simulink model "CRTsfun"  (Simulink 8.0)
settings: Solver=ode45  StartTime=0.0  StopTime=10.0  RelTol=1e-3
undefined symbols (not defined in the file or in its folder): vicrt_initcallback, vicrt_initmexcallback, vicrt_inputfile, vicrt_simulationmanager
(part 1 of 3)
settings Model: Creator=battags  LastModifiedBy=battags

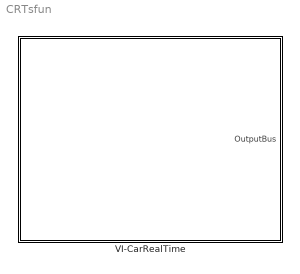
== system CRTsfun ==
  VI-CarRealTime : Subsystem  InitFcn=vicrt_simulationmanager(0);
      mask help: Full VI-CarRealTime mex integrated with IO Bus
      settings: CopyFcn=set_param(gcb, 'LinkStatus', 'none');  ModelCloseFcn=vicrt_simulationmanager(2);  OpenFcn=vicrt_simulationmanager(1);
      mask Display: image(imread('vehicle.jpg'));color('red');port_label('output',1,'OutputBus');

== system CRTsfun/VI-CarRealTime ==
  Input_Bus : Subsystem  LoadFcn=vicrt_initcallback(gcb);
      settings: CopyFcn=vicrt_initcallback(gcb);
  Output_Bus : Subsystem  Description=Outputs
      settings: CopyFcn=%set_param(gcb, 'LinkStatus', 'none')
  vicrt_mex Standard : Subsystem  mask{vicrt_inputfile=vicrt_inputfile, vicrt_outprefix='', intStep=0.001, AniFlag=off, inpPortDim=225, outPortDim=1100}
      mask prompts: vicrt_inputfile "VI-CarRealtime input file"; vicrt_outprefix "VI-CarRealTime output prefix"; intStep "Integration step"; AniFlag "live animation"; inpPortDim "input port dimension"; outPortDim "output port dimension"
      mask init:
      | custDriv=[1,1,1];
      settings: CopyFcn=set_param(gcb, 'LinkStatus', 'none')
  OutputBus : Outport
  wires:
  Output_Bus/1(OutputBus) -> OutputBus/1
  Input_Bus/1(vicrt input) -> vicrt_mex Standard/1(In1)
  vicrt_mex Standard/1(Out1) -> Output_Bus/1(Outputs)

== system CRTsfun/VI-CarRealTime/Input_Bus ==
  Bus2Map : Subsystem
  Inputs : Subsystem
  Standard_Input_Bus : Constant
  VicrtBusAssignment : BusAssignment  AssignedSignals=Standard_Input_Bus
  vicrt input : Outport
  wires:
  Standard_Input_Bus/1 -> VicrtBusAssignment/2
  Inputs/1(Inputs) -> VicrtBusAssignment/1  "Inputs"
  VicrtBusAssignment/1 -> Bus2Map/1(Bus In)
  Bus2Map/1(Map Out) -> vicrt input/1

== system CRTsfun/VI-CarRealTime/Output_Bus ==
  Outputs : Inport
  IOmap2bus : Subsystem
  VicrtBusSelector : BusSelector  InitFcn=warning('off','Simulink:blocks:BusSelectorDuplicateLeafSignalInMuxedOutput');  StartFcn=warning('on','Simulink:blocks:BusSelectorDuplicateLeafSignalInMuxedOutput');  OutputSignals=aero_forces  OutputAsBus=on
  adapter : Subsystem
  OutputBus : Outport
  wires:
  adapter/1(outputBus) -> OutputBus/1
  VicrtBusSelector/1 -> adapter/1(inputBus)
  Outputs/1 -> IOmap2bus/1(In)
  IOmap2bus/1(Out) -> VicrtBusSelector/1

== system CRTsfun/VI-CarRealTime/vicrt_mex Standard ==
  In1 : Inport
  vicrt_mex : S-Function  InitFcn=vicrt_initmexcallback(gcb);  FunctionName=vicrt_mex  Parameters=vicrt_inputfile,vicrt_outprefix,AniFlag,intStep,inpPortDim,outPortDim  EnableBusSupport=off
  Out1 : Outport
  wires:
  In1/1 -> vicrt_mex/1
  vicrt_mex/1 -> Out1/1

== system CRTsfun/VI-CarRealTime/Input_Bus/Bus2Map ==
  Bus In : Inport
  Bus Selector : BusSelector  OutputSignals=Driver_Demands.str_swa,Driver_Demands.throttle,Driver_Demands.gear,Driver_Demands.clutch,Driver_Demands.brake,Driver_Demands.rack_displacement,Brake_System_General.brk_mast_cyl_pres,Brake_System_General.brk_bias_front,Driver_Demands.user_maneuver_ID,Friction.tire_mu.L1,Friction.tire_mu.L2,Friction.tire_mu.R1,Friction.tire_mu.R2,Subsystem_Activation.Internal_Brake_System_Activity.L1,Brake_System.brk_mmag_sign.L1,Brake_System.brk_mmag_unsign.L1,Brake_System.brk_pres.L1,Brake_System.brk_pres_gain.L1,Brake_System.brk_mu.L1,Subsystem_Activation.Internal_Brake_System_Activity.L2,Brake_System.brk_mmag_sign.L2,Brake_System.brk_mmag_unsign.L2,Brake_System.brk_pres.L2,Brake_System.brk_pres_gain.L2,Brake_System.brk_mu.L2,Subsystem_Activation.Internal_Brake_System_Activity.R1,Brake_System.brk_mmag_sign.R1,Brake_System.brk_mmag_unsign.R1,Brake_System.brk_pres.R1,Brake_System.brk_pres_gain.R1,Brake_System.brk_mu.R1,Subsystem_Activation.Internal_Brake_System_Activity.R2,Brake_System.brk_mmag_sign.R2,Brake_System.brk_mmag_unsign.R2,Brake_System.brk_pres.R2,Brake_System.brk_pres_gain.R2,Brake_System.brk_mu.R2,Hook.Fx.rear,Hook.Fy.rear,Hook.Fz.rear,Hook.Mx.rear,Hook.My.rear,Hook.Mz.rear,Rear_Steering_Actuator_disp.str_swa.left,Rear_Steering_Actuator_disp.str_swa.right,Steering.steer_at_spindle.L1,Steering.steer_at_spindle.L2,Steering.steer_at_spindle.R1,Steering.steer_at_spindle.R2,Subsystem_Activation.Internal_Clutch_Activity,Subsystem_Activation.Internal_Engine_Activity,Subsystem_Activation.Internal_Gearbox_Activity,Engine.engine_omega,Engine.engine_max_trq,Engine.engine_min_trq,Engine.engine_trq,Engine.non_termic_engine_trq,GearBox.transmission_ratio,Clutch.clutch_trq,Clutch.clutch_slip_angle,Antiroll_Bar.activity_flag.front,Antiroll_Bar.activity_flag.rear,Antiroll_Bar.force.front,Antiroll_Bar.force.rear,Subsystem_Activation.Internal_Aero_Activity,Aerodynamic.fx_front,Aerodynamic.fy_front,Aerodynamic.fz_front,Aerodynamic.fx_rear,Aerodynamic.fy_rear,Aerodynamic.fz_rear,Aerodynamic.fx_center,Aerodynamic.fy_center,Aerodynamic.fz_center,Aerodynamic.mx,Aerodynamic.my,Aerodynamic.mz,Irregularity.road.L1,Irregularity.road.L2,Irregularity.road.R1,Irregularity.road.R2,Main_Damper.force.L1,Main_Damper.activity_flag.L1,Main_Damper.force.L2,Main_Damper.activity_flag.L2,Main_Damper.force.R1,Main_Damper.activity_flag.R1,Main_Damper.force.R2,Main_Damper.activity_flag.R2,Main_Spring.force.L1,Main_Spring.activity_flag.L1,Main_Spring.force.L2,Main_Spring.activity_flag.L2,Main_Spring.force.R1,Main_Spring.activity_flag.R1,Main_Spring.force.R2,Main_Spring.activity_flag.R2,Main_Bumpstop.force.L1,Main_Bumpstop.activity_flag.L1,Main_Bumpstop.force.L2,Main_Bumpstop.activity_flag.L2,Main_Bumpstop.force.R1,Main_Bumpstop.activity_flag.R1,Main_Bumpstop.force.R2,Main_Bumpstop.activity_flag.R2,Main_Reboundstop.force.L1,Main_Reboundstop.activity_flag.L1,Main_Reboundstop.force.L2,Main_Reboundstop.activity_flag.L2,Main_Reboundstop.force.R1,Main_Reboundstop.activity_flag.R1,Main_Reboundstop.force.R2,Main_Reboundstop.activity_flag.R2,Auxiliary_vertical.force.L1,Auxiliary_vertical.activity_flag.L1,Auxiliary_vertical.force.L2,Auxiliary_vertical.activity_flag.L2,Auxiliary_vertical.force.R1,Auxiliary_vertical.activity_flag.R1,Auxiliary_vertical.force.R2,Auxiliary_vertical.activity_flag.R2,Third_Element.Damper_force.front,Third_Element.Damper_activity_flag.front,Third_Element.Damper_force.rear,Third_Element.Damper_activity_flag.rear,Third_Element.Spring.front,Third_Element.Spring_activity_flag.front,Third_Element.Spring.rear,Third_Element.Spring_activity_flag.rear,Mono_Element.Damper.front,Mono_Element.Damper_activity_flag.front,Mono_Element.Damper.rear,Mono_Element.Damper_activity_flag.rear,Mono_Element.Inerter.front,Mono_Element.Inerter_activity_flag.front,Mono_Element.Inerter.rear,Mono_Element.Inerter_activity_flag.rear,Mono_Element.Spring.front,Mono_Element.Spring_activity_flag.front,Mono_Element.Spring.rear,Mono_Element.Spring_activity_flag.rear,Mono_Element.Bumpstop_Spring.front,Mono_Element.Bumpstop_Spring_activity_flag.front,Mono_Element.Bumpstop_Spring.rear,Mono_Element.Bumpstop_Spring_activity_flag.rear,Mono_Element.Reboundstop_Spring.front,Mono_Element.Reboundstop_Spring_activity_flag.front,Mono_Element.Reboundstop_Spring.rear,Mono_Element.Reboundstop_Spring_activity_flag.rear,Mono_Element.Bumpstop_Damper.front,Mono_Element.Bumpstop_Damper_activity_flag.front,Mono_Element.Bumpstop_Damper.rear,Mono_Element.Bumpstop_Damper_activity_flag.rear,Mono_Element.Reboundstop_Damper.front,Mono_Element.Reboundstop_Damper_activity_flag.front,Mono_Element.Reboundstop_Damper.rear,Mono_Element.Reboundstop_Damper_activity_flag.rear,Subsystem_Activation.Tire_Force_x.L1,Subsystem_Activation.Tire_Force_y.L1,Subsystem_Activation.Tire_Force_z.L1,Subsystem_Activation.Tire_Moment_x.L1,Subsystem_Activation.Tire_Moment_y.L1,Subsystem_Activation.Tire_Moment_z.L1,Tire_Force.Fx.L1,Tire_Force.Fy.L1,Tire_Force.Fz.L1,Tire_Moment.Mx.L1,Tire_Moment.My.L1,Tire_Moment.Mz.L1,Subsystem_Activation.Tire_Force_x.L2,Subsystem_Activation.Tire_Force_y.L2,Subsystem_Activation.Tire_Force_z.L2,Subsystem_Activation.Tire_Moment_x.L2,Subsystem_Activation.Tire_Moment_y.L2,Subsystem_Activation.Tire_Moment_z.L2,Tire_Force.Fx.L2,Tire_Force.Fy.L2,Tire_Force.Fz.L2,Tire_Moment.Mx.L2,Tire_Moment.My.L2,Tire_Moment.Mz.L2,Subsystem_Activation.Tire_Force_x.R1,Subsystem_Activation.Tire_Force_y.R1,Subsystem_Activation.Tire_Force_z.R1,Subsystem_Activation.Tire_Moment_x.R1,Subsystem_Activation.Tire_Moment_y.R1,Subsystem_Activation.Tire_Moment_z.R1,Tire_Force.Fx.R1,Tire_Force.Fy.R1,Tire_Force.Fz.R1,Tire_Moment.Mx.R1,Tire_Moment.My.R1,Tire_Moment.Mz.R1,Subsystem_Activation.Tire_Force_x.R2,Subsystem_Activation.Tire_Force_y.R2,Subsystem_Activation.Tire_Force_z.R2,Subsystem_Activation.Tire_Moment_x.R2,Subsystem_Activation.Tire_Moment_y.R2,Subsystem_Activation.Tire_Moment_z.R2,Tire_Force.Fx.R2,Tire_Force.Fy.R2,Tire_Force.Fz.R2,Tire_Moment.Mx.R2,Tire_Moment.My.R2,Tire_Moment.Mz.R2,Wheel_driving.moment.L1,Wheel_driving.moment.L2,Wheel_driving.moment.R1,Wheel_driving.moment.R2,Ext_Body.force.X,Ext_Body.force.Y,Ext_Body.force.Z,Ext_Body.moment.X,Ext_Body.moment.Y,Ext_Body.moment.Z,Ext_Ground.force.X,Ext_Ground.force.Y,Ext_Ground.force.Z,Ext_Ground.moment.X,Ext_Ground.moment.Y,Ext_Ground.moment.Z,Ext_Tracking.force.X,Ext_Tracking.force.Y,Ext_Tracking.moment.X,Ext_Tracking.moment.Y
  Mux : Mux  Inputs=225
  Map Out : Outport
  wires:
  Bus Selector/225 -> Mux/225  "<Y>"
  Bus Selector/224 -> Mux/224  "<X>"
  Bus Selector/223 -> Mux/223  "<Y>"
  Bus Selector/222 -> Mux/222  "<X>"
  Bus Selector/221 -> Mux/221  "<Z>"
  Bus Selector/220 -> Mux/220  "<Y>"
  Bus Selector/219 -> Mux/219  "<X>"
  Bus Selector/218 -> Mux/218  "<Z>"
  Bus Selector/217 -> Mux/217  "<Y>"
  Bus Selector/216 -> Mux/216  "<X>"
  Bus Selector/215 -> Mux/215  "<Z>"
  Bus Selector/214 -> Mux/214  "<Y>"
  Bus Selector/213 -> Mux/213  "<X>"
  Bus Selector/212 -> Mux/212  "<Z>"
  Bus Selector/211 -> Mux/211  "<Y>"
  Bus Selector/210 -> Mux/210  "<X>"
  Bus Selector/209 -> Mux/209  "<R2>"
  Bus Selector/208 -> Mux/208  "<R1>"
  Bus Selector/207 -> Mux/207  "<L2>"
  Bus Selector/206 -> Mux/206  "<L1>"
  Bus Selector/205 -> Mux/205  "<R2>"
  Bus Selector/204 -> Mux/204  "<R2>"
  Bus Selector/203 -> Mux/203  "<R2>"
  Bus Selector/202 -> Mux/202  "<R2>"
  Bus Selector/201 -> Mux/201  "<R2>"
  Bus Selector/200 -> Mux/200  "<R2>"
  Bus Selector/199 -> Mux/199  "<R2>"
  Bus Selector/198 -> Mux/198  "<R2>"
  Bus Selector/197 -> Mux/197  "<R2>"
  Bus Selector/196 -> Mux/196  "<R2>"
  Bus Selector/195 -> Mux/195  "<R2>"
  Bus Selector/194 -> Mux/194  "<R2>"
  Bus Selector/193 -> Mux/193  "<R1>"
  Bus Selector/192 -> Mux/192  "<R1>"
  Bus Selector/191 -> Mux/191  "<R1>"
  Bus Selector/190 -> Mux/190  "<R1>"
  Bus Selector/189 -> Mux/189  "<R1>"
  Bus Selector/188 -> Mux/188  "<R1>"
  Bus Selector/187 -> Mux/187  "<R1>"
  Bus Selector/186 -> Mux/186  "<R1>"
  Bus Selector/185 -> Mux/185  "<R1>"
  Bus Selector/184 -> Mux/184  "<R1>"
  Bus Selector/183 -> Mux/183  "<R1>"
  Bus Selector/182 -> Mux/182  "<R1>"
  Bus Selector/181 -> Mux/181  "<L2>"
  Bus Selector/180 -> Mux/180  "<L2>"
  Bus Selector/179 -> Mux/179  "<L2>"
  Bus Selector/178 -> Mux/178  "<L2>"
  Bus Selector/177 -> Mux/177  "<L2>"
  Bus Selector/176 -> Mux/176  "<L2>"
  Bus Selector/175 -> Mux/175  "<L2>"
  Bus Selector/174 -> Mux/174  "<L2>"
  Bus Selector/173 -> Mux/173  "<L2>"
  Bus Selector/172 -> Mux/172  "<L2>"
  Bus Selector/171 -> Mux/171  "<L2>"
  Bus Selector/170 -> Mux/170  "<L2>"
  Bus Selector/169 -> Mux/169  "<L1>"
  Bus Selector/168 -> Mux/168  "<L1>"
  Bus Selector/167 -> Mux/167  "<L1>"
  Bus Selector/166 -> Mux/166  "<L1>"
  Bus Selector/165 -> Mux/165  "<L1>"
  Bus Selector/164 -> Mux/164  "<L1>"
  Bus Selector/163 -> Mux/163  "<L1>"
  Bus Selector/162 -> Mux/162  "<L1>"
  Bus Selector/161 -> Mux/161  "<L1>"
  Bus Selector/160 -> Mux/160  "<L1>"
  Bus Selector/159 -> Mux/159  "<L1>"
  Bus Selector/158 -> Mux/158  "<L1>"
  Bus Selector/157 -> Mux/157  "<rear>"
  Bus Selector/156 -> Mux/156  "<rear>"
  Bus Selector/155 -> Mux/155  "<front>"
  Bus Selector/154 -> Mux/154  "<front>"
  Bus Selector/153 -> Mux/153  "<rear>"
  Bus Selector/152 -> Mux/152  "<rear>"
  Bus Selector/151 -> Mux/151  "<front>"
  Bus Selector/150 -> Mux/150  "<front>"
  Bus Selector/149 -> Mux/149  "<rear>"
  Bus Selector/148 -> Mux/148  "<rear>"
  Bus Selector/147 -> Mux/147  "<front>"
  Bus Selector/146 -> Mux/146  "<front>"
  Bus Selector/145 -> Mux/145  "<rear>"
  Bus Selector/144 -> Mux/144  "<rear>"
  Bus Selector/143 -> Mux/143  "<front>"
  Bus Selector/142 -> Mux/142  "<front>"
  Bus Selector/141 -> Mux/141  "<rear>"
  Bus Selector/140 -> Mux/140  "<rear>"
  Bus Selector/139 -> Mux/139  "<front>"
  Bus Selector/138 -> Mux/138  "<front>"
  Bus Selector/137 -> Mux/137  "<rear>"
  Bus Selector/136 -> Mux/136  "<rear>"
  Bus Selector/135 -> Mux/135  "<front>"
  Bus Selector/134 -> Mux/134  "<front>"
  Bus Selector/133 -> Mux/133  "<rear>"
  Bus Selector/132 -> Mux/132  "<rear>"
  Bus Selector/131 -> Mux/131  "<front>"
  Bus Selector/130 -> Mux/130  "<front>"
  Bus Selector/129 -> Mux/129  "<rear>"
  Bus Selector/128 -> Mux/128  "<rear>"
  Bus Selector/127 -> Mux/127  "<front>"
  Bus Selector/126 -> Mux/126  "<front>"
  Bus Selector/125 -> Mux/125  "<rear>"
  Bus Selector/124 -> Mux/124  "<rear>"
  Bus Selector/123 -> Mux/123  "<front>"
  Bus Selector/122 -> Mux/122  "<front>"
  Bus Selector/121 -> Mux/121  "<R2>"
  Bus Selector/120 -> Mux/120  "<R2>"
  Bus Selector/119 -> Mux/119  "<R1>"
  Bus Selector/118 -> Mux/118  "<R1>"
  Bus Selector/117 -> Mux/117  "<L2>"
  Bus Selector/116 -> Mux/116  "<L2>"
  Bus Selector/115 -> Mux/115  "<L1>"
  Bus Selector/114 -> Mux/114  "<L1>"
  Bus Selector/113 -> Mux/113  "<R2>"
  Bus Selector/112 -> Mux/112  "<R2>"
  Bus Selector/111 -> Mux/111  "<R1>"
  Bus Selector/110 -> Mux/110  "<R1>"
  Bus Selector/109 -> Mux/109  "<L2>"
  Bus Selector/108 -> Mux/108  "<L2>"
  Bus Selector/107 -> Mux/107  "<L1>"
  Bus Selector/106 -> Mux/106  "<L1>"
  Bus Selector/105 -> Mux/105  "<R2>"
  Bus Selector/104 -> Mux/104  "<R2>"
  Bus Selector/103 -> Mux/103  "<R1>"
  Bus Selector/102 -> Mux/102  "<R1>"
  Bus Selector/101 -> Mux/101  "<L2>"
  Bus Selector/100 -> Mux/100  "<L2>"
  Bus Selector/99 -> Mux/99  "<L1>"
  Bus Selector/98 -> Mux/98  "<L1>"
  Bus Selector/97 -> Mux/97  "<R2>"
  Bus Selector/96 -> Mux/96  "<R2>"
  Bus Selector/95 -> Mux/95  "<R1>"
  Bus Selector/94 -> Mux/94  "<R1>"
  Bus Selector/93 -> Mux/93  "<L2>"
  Bus Selector/92 -> Mux/92  "<L2>"
  Bus Selector/91 -> Mux/91  "<L1>"
  Bus Selector/90 -> Mux/90  "<L1>"
  Bus Selector/89 -> Mux/89  "<R2>"
  Bus Selector/88 -> Mux/88  "<R2>"
  Bus Selector/87 -> Mux/87  "<R1>"
  Bus Selector/86 -> Mux/86  "<R1>"
  Bus Selector/85 -> Mux/85  "<L2>"
  Bus Selector/84 -> Mux/84  "<L2>"
  Bus Selector/83 -> Mux/83  "<L1>"
  Bus Selector/82 -> Mux/82  "<L1>"
  Bus Selector/81 -> Mux/81  "<R2>"
  Bus Selector/80 -> Mux/80  "<R1>"
  Bus Selector/79 -> Mux/79  "<L2>"
  Bus Selector/78 -> Mux/78  "<L1>"
  Bus Selector/77 -> Mux/77  "<mz>"
  Bus Selector/76 -> Mux/76  "<my>"
  Bus Selector/75 -> Mux/75  "<mx>"
  Bus Selector/74 -> Mux/74  "<fz_center>"
  Bus Selector/73 -> Mux/73  "<fy_center>"
  Bus Selector/72 -> Mux/72  "<fx_center>"
  Bus Selector/71 -> Mux/71  "<fz_rear>"
  Bus Selector/70 -> Mux/70  "<fy_rear>"
  Bus Selector/69 -> Mux/69  "<fx_rear>"
  Bus Selector/68 -> Mux/68  "<fz_front>"
  Bus Selector/67 -> Mux/67  "<fy_front>"
  Bus Selector/66 -> Mux/66  "<fx_front>"
  Bus Selector/65 -> Mux/65  "<Internal_Aero_Activity>"
  Bus Selector/64 -> Mux/64  "<rear>"
  Bus Selector/63 -> Mux/63  "<front>"
  Bus Selector/62 -> Mux/62  "<rear>"
  Bus Selector/61 -> Mux/61  "<front>"
  Bus Selector/60 -> Mux/60  "<clutch_slip_angle>"
  Bus Selector/59 -> Mux/59  "<clutch_trq>"
  Bus Selector/58 -> Mux/58  "<transmission_ratio>"
  Bus Selector/57 -> Mux/57  "<non_termic_engine_trq>"
  Bus Selector/56 -> Mux/56  "<engine_trq>"
  Bus Selector/55 -> Mux/55  "<engine_min_trq>"
  Bus Selector/54 -> Mux/54  "<engine_max_trq>"
  Bus Selector/53 -> Mux/53  "<engine_omega>"
  Bus Selector/52 -> Mux/52  "<Internal_Gearbox_Activity>"
  Bus Selector/51 -> Mux/51  "<Internal_Engine_Activity>"
  Bus Selector/50 -> Mux/50  "<Internal_Clutch_Activity>"
  Bus Selector/49 -> Mux/49  "<R2>"
  Bus Selector/48 -> Mux/48  "<R1>"
  Bus Selector/47 -> Mux/47  "<L2>"
  Bus Selector/46 -> Mux/46  "<L1>"
  Bus Selector/45 -> Mux/45  "<right>"
  Bus Selector/44 -> Mux/44  "<left>"
  Bus Selector/43 -> Mux/43  "<rear>"
  Bus Selector/42 -> Mux/42  "<rear>"
  Bus Selector/41 -> Mux/41  "<rear>"
  Bus Selector/40 -> Mux/40  "<rear>"
  Bus Selector/39 -> Mux/39  "<rear>"
  Bus Selector/38 -> Mux/38  "<rear>"
  Bus Selector/37 -> Mux/37  "<R2>"
  Bus Selector/36 -> Mux/36  "<R2>"
  Bus Selector/35 -> Mux/35  "<R2>"
  Bus Selector/34 -> Mux/34  "<R2>"
  Bus Selector/33 -> Mux/33  "<R2>"
  Bus Selector/32 -> Mux/32  "<R2>"
  Bus Selector/31 -> Mux/31  "<R1>"
  Bus Selector/30 -> Mux/30  "<R1>"
  Bus Selector/29 -> Mux/29  "<R1>"
  Bus Selector/28 -> Mux/28  "<R1>"
  Bus Selector/27 -> Mux/27  "<R1>"
  Bus Selector/26 -> Mux/26  "<R1>"
  Bus Selector/25 -> Mux/25  "<L2>"
  Bus Selector/24 -> Mux/24  "<L2>"
  Bus Selector/23 -> Mux/23  "<L2>"
  Bus Selector/22 -> Mux/22  "<L2>"
  Bus Selector/21 -> Mux/21  "<L2>"
  Bus Selector/20 -> Mux/20  "<L2>"
  Bus Selector/19 -> Mux/19  "<L1>"
  Bus Selector/18 -> Mux/18  "<L1>"
  Bus Selector/17 -> Mux/17  "<L1>"
  Bus Selector/16 -> Mux/16  "<L1>"
  Bus Selector/15 -> Mux/15  "<L1>"
  Bus Selector/14 -> Mux/14  "<L1>"
  Bus Selector/13 -> Mux/13  "<R2>"
  Bus Selector/12 -> Mux/12  "<R1>"
  Bus Selector/11 -> Mux/11  "<L2>"
  Bus Selector/10 -> Mux/10  "<L1>"
  Bus Selector/9 -> Mux/9  "<user_maneuver_ID>"
  Bus Selector/8 -> Mux/8  "<brk_bias_front>"
  Bus Selector/7 -> Mux/7  "<brk_mast_cyl_pres>"
  Bus Selector/6 -> Mux/6  "<rack_displacement>"
  Bus Selector/5 -> Mux/5  "<brake>"
  Bus Selector/4 -> Mux/4  "<clutch>"
  Bus Selector/3 -> Mux/3  "<gear>"
  Bus Selector/2 -> Mux/2  "<throttle>"
  Bus Selector/1 -> Mux/1  "<str_swa>"
  Bus In/1 -> Bus Selector/1
  Mux/1 -> Map Out/1

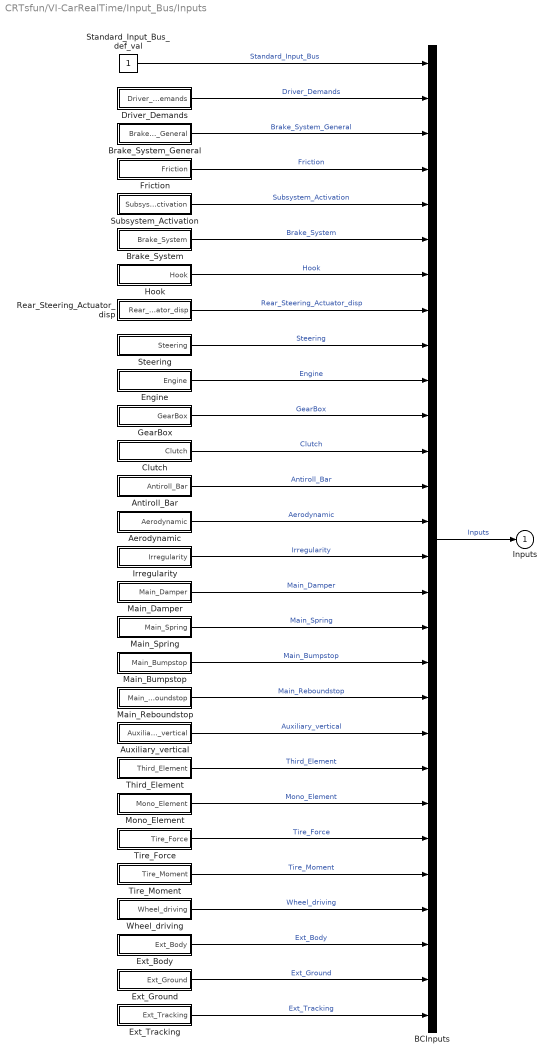
== system CRTsfun/VI-CarRealTime/Input_Bus/Inputs ==
  Aerodynamic : Subsystem
  Antiroll_Bar : Subsystem
  Auxiliary_vertical : Subsystem
  BCInputs : BusCreator  Inputs=28
  Brake_System : Subsystem
  Brake_System_General : Subsystem
  Clutch : Subsystem
  Driver_Demands : Subsystem
  Engine : Subsystem
  Ext_Body : Subsystem
  Ext_Ground : Subsystem
  Ext_Tracking : Subsystem
  Friction : Subsystem
  GearBox : Subsystem
  Hook : Subsystem
  Irregularity : Subsystem
  Main_Bumpstop : Subsystem
  Main_Damper : Subsystem
  Main_Reboundstop : Subsystem
  Main_Spring : Subsystem
  Mono_Element : Subsystem
  Rear_Steering_Actuator_disp : Subsystem
  Standard_Input_Bus_def_val : Constant
  Steering : Subsystem
  Subsystem_Activation : Subsystem
  Third_Element : Subsystem
  Tire_Force : Subsystem
  Tire_Moment : Subsystem
  Wheel_driving : Subsystem
  Inputs : Outport
  wires:
  Ext_Tracking/1(Ext_Tracking) -> BCInputs/28  "Ext_Tracking"
  Ext_Ground/1(Ext_Ground) -> BCInputs/27  "Ext_Ground"
  Ext_Body/1(Ext_Body) -> BCInputs/26  "Ext_Body"
  Wheel_driving/1(Wheel_driving) -> BCInputs/25  "Wheel_driving"
  Tire_Moment/1(Tire_Moment) -> BCInputs/24  "Tire_Moment"
  Tire_Force/1(Tire_Force) -> BCInputs/23  "Tire_Force"
  Mono_Element/1(Mono_Element) -> BCInputs/22  "Mono_Element"
  Third_Element/1(Third_Element) -> BCInputs/21  "Third_Element"
  Auxiliary_vertical/1(Auxiliary_vertical) -> BCInputs/20  "Auxiliary_vertical"
  Main_Reboundstop/1(Main_Reboundstop) -> BCInputs/19  "Main_Reboundstop"
  Main_Bumpstop/1(Main_Bumpstop) -> BCInputs/18  "Main_Bumpstop"
  Main_Spring/1(Main_Spring) -> BCInputs/17  "Main_Spring"
  Main_Damper/1(Main_Damper) -> BCInputs/16  "Main_Damper"
  Irregularity/1(Irregularity) -> BCInputs/15  "Irregularity"
  Aerodynamic/1(Aerodynamic) -> BCInputs/14  "Aerodynamic"
  Antiroll_Bar/1(Antiroll_Bar) -> BCInputs/13  "Antiroll_Bar"
  Clutch/1(Clutch) -> BCInputs/12  "Clutch"
  GearBox/1(GearBox) -> BCInputs/11  "GearBox"
  Engine/1(Engine) -> BCInputs/10  "Engine"
  Steering/1(Steering) -> BCInputs/9  "Steering"
  Rear_Steering_Actuator_disp/1(Rear_Steering_Actuator_disp) -> BCInputs/8  "Rear_Steering_Actuator_disp"
  Hook/1(Hook) -> BCInputs/7  "Hook"
  Brake_System/1(Brake_System) -> BCInputs/6  "Brake_System"
  Subsystem_Activation/1(Subsystem_Activation) -> BCInputs/5  "Subsystem_Activation"
  Friction/1(Friction) -> BCInputs/4  "Friction"
  Brake_System_General/1(Brake_System_General) -> BCInputs/3  "Brake_System_General"
  Driver_Demands/1(Driver_Demands) -> BCInputs/2  "Driver_Demands"
  Standard_Input_Bus_def_val/1 -> BCInputs/1  "Standard_Input_Bus"
  BCInputs/1 -> Inputs/1  "Inputs"
